simulink model "Final_Project_2"  (R2023b)
settings: Solver=FixedStepAuto  StartTime=0.0  StopTime=inf  FixedStep=0.01  RelTol=1e-3  EnableMultiTasking=on
libraries: arduinolib x8, arduinosensorlib x1
settings Model: ExtModeTrigDuration=2  Creator=FM23  LastModifiedBy=FM23
settings OptimizationCC: EnhancedBackFolding=on  PassReuseOutputArgsAs=Individual arguments  ZeroExternalMemoryAtStartup=off  ZeroInternalMemoryAtStartup=off  MaxStackSize=64  OptimizeBlockOrder=speed  DifferentSizesBufferReuse=on  OptimizationCustomize=off  EfficientTunableParamExpr=on
settings DebuggingCC: ParameterTunabilityLossMsg=error
settings HardwareCC: ProdBitPerInt=16  ProdBitPerPointer=16  ProdBitPerSizeT=16  ProdBitPerPtrDiffT=16  ProdLargestAtomicFloat=None  ProdWordSize=8  ProdHWDeviceType=Atmel->AVR
settings SFSimCC: MATLABDynamicMemAlloc=off
settings RTWCC: Description=Embedded Coder  SystemTargetFile=ert.tlc  HardwareBoard=Arduino Mega 2560  TemplateMakefile=ert_default_tmf  Toolchain=Arduino AVR  BuildConfiguration=Faster Runs
settings CodeAppCC: ForceParamTrailComments=on  IgnoreCustomStorageClasses=off  OperatorAnnotations=on  SimulinkDataObjDesc=on  SFDataObjDesc=on  InsertBlockDesc=on
settings ERTTargetCC: SupportContinuousTime=on  SupportVariableSizeSignals=on  ExtModeTransport=3  ExtModeStaticAlloc=on  ExtModeAutomaticAllocSize=off  ExtModeStaticAllocSize=2048  ExtModeMexFile=ext_xcp  ExtModeIntrfLevel=Level2 - Open

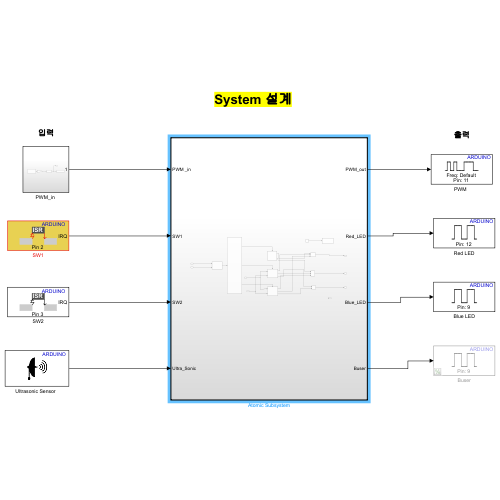
[thumbnail: Simulink's stored preview of the top-level diagram]
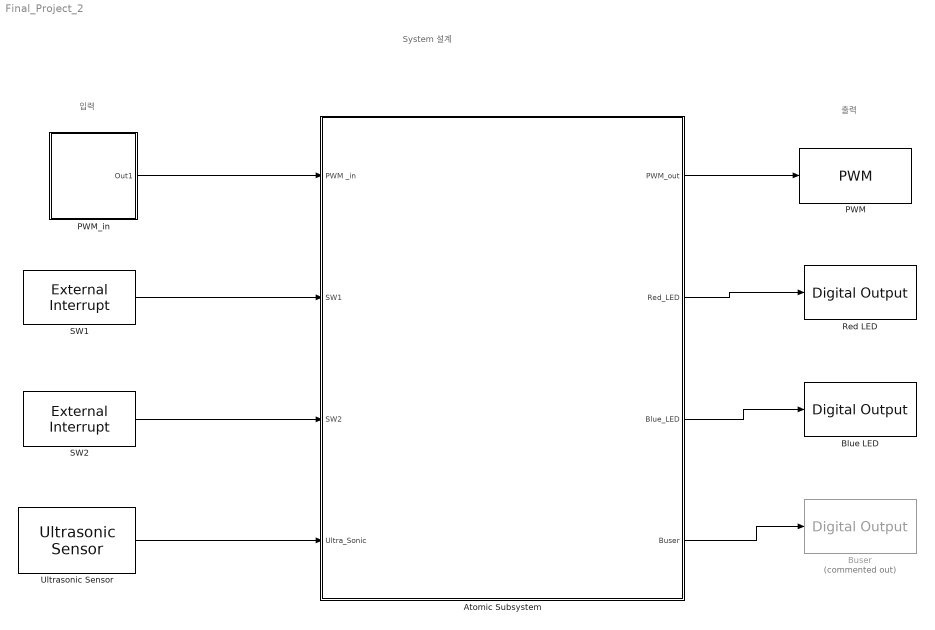
== system Final_Project_2 ==
  note: System 설계
  note: 입력
  note: 출력
  Atomic Subsystem : Subsystem  TreatAsAtomicUnit=on
  Blue LED : arduinolib/Digital Output  pinNumber=9  Direction=output  blockPlatform=arduino
  Buser : arduinolib/Digital Output  Commented=on  pinNumber=9  Direction=output  blockPlatform=arduino
  "PWM  " : arduinolib/PWM  pinNumber=11  frequencyType=Default  desiredFrequency=490.2  achievableFrequency=490.2
  "PWM_in " : Subsystem
  Red LED : arduinolib/Digital Output  pinNumber=12  Direction=output  blockPlatform=arduino
  SW1 : arduinolib/External Interrupt  Pin=2  PullUp=off  Mode=RISING  InterruptSimulationInput=off
  SW2 : arduinolib/External Interrupt  Pin=3  PullUp=off  Mode=RISING  InterruptSimulationInput=off
  "Ultrasonic Sensor  " : arduinosensorlib/Ultrasonic Sensor  NumSignalPins=2  TrigPin=50  EchoPin=51  SignalPin=3  SampleTime_=0.1  blockPlatform=ARDUINO
  wires:
  "Ultrasonic Sensor  "/1 -> Atomic Subsystem/4(Ultra_Sonic)
  "PWM_in "/1(Out1) -> Atomic Subsystem/1(PWM _in)
  Atomic Subsystem/1(" PWM_out") -> "PWM  "/1
  Atomic Subsystem/2(Red_LED) -> Red LED/1
  Atomic Subsystem/3(Blue_LED) -> Blue LED/1
  Atomic Subsystem/4(Buser) -> Buser/1
  SW1/1 -> Atomic Subsystem/2(SW1)
  SW2/1 -> Atomic Subsystem/3(SW2)

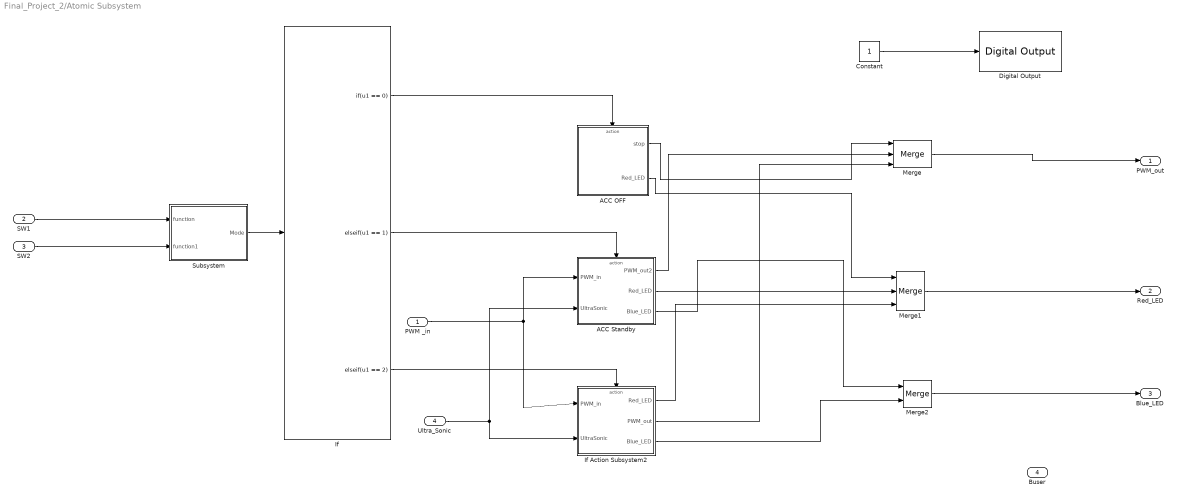
== system Final_Project_2/Atomic Subsystem ==
  PWM _in : Inport
  SW1 : Inport  Port=2
  SW2 : Inport  Port=3
  Ultra_Sonic : Inport  Port=4
  ACC OFF : Subsystem  TreatAsAtomicUnit=on
  "ACC Standby   " : Subsystem  TreatAsAtomicUnit=on
  Constant : Constant
  Digital Output : arduinolib/Digital Output  pinNumber=13  Direction=output  blockPlatform=arduino
  If : If  IfExpression=u1 == 0  ElseIfExpressions=u1 == 1, u1 == 2  ShowElse=off
  If Action Subsystem2 : Subsystem  TreatAsAtomicUnit=on
  Merge : Merge  Inputs=3
  Merge1 : Merge  Inputs=3
  Merge2 : Merge
  Subsystem : Subsystem
  " PWM_out" : Outport
  Red_LED : Outport  Port=2
  Blue_LED : Outport  Port=3
  Buser : Outport  Port=4
  wires:
  Merge1/1 -> Red_LED/1
  Merge2/1 -> Blue_LED/1
  Merge/1 -> " PWM_out"/1
  If/1 -> ACC OFF/Action
  PWM _in/1 -> If Action Subsystem2/1(PWM_in), "ACC Standby   "/1(PWM_in)
  If/2 -> "ACC Standby   "/Action
  ACC OFF/1(stop) -> Merge/1
  If/3 -> If Action Subsystem2/Action
  ACC OFF/2(Red_LED) -> Merge1/1
  "ACC Standby   "/2(Red_LED) -> Merge1/2
  "ACC Standby   "/3(Blue_LED) -> Merge2/1
  "ACC Standby   "/1(PWM_out2) -> Merge/2
  Ultra_Sonic/1 -> If Action Subsystem2/2(UltraSonic), "ACC Standby   "/2(UltraSonic)
  If Action Subsystem2/2(PWM_out) -> Merge/3
  If Action Subsystem2/1(Red_LED) -> Merge1/3
  If Action Subsystem2/3(Blue_LED) -> Merge2/2
  Constant/1 -> Digital Output/1
  Subsystem/1(Mode) -> If/1
  SW1/1 -> Subsystem/1(function)
  SW2/1 -> Subsystem/2(function1)

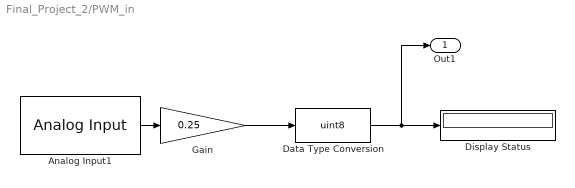
== system Final_Project_2/PWM_in  ==
  Analog Input1 : arduinolib/Analog Input  pinNumber=4  ReadResultsOnly=off  ConversionTriggerSource=Software  ExternalTriggerType=uint32( 0 )  OutputDataType=uint16  EnableConversionCompleteNotify=off  EnableOuputStatus=off  SampleTime=-1  blockPlatform=arduino
  Data Type Conversion : DataTypeConversion  OutDataTypeStr=uint8  SaturateOnIntegerOverflow=off  RndMeth=Floor
  Display Status : Display
  Gain : Gain  Gain=0.25
  Out1 : Outport
  wires:
  Analog Input1/1 -> Gain/1
  Gain/1 -> Data Type Conversion/1
  Data Type Conversion/1 -> Out1/1, Display Status/1

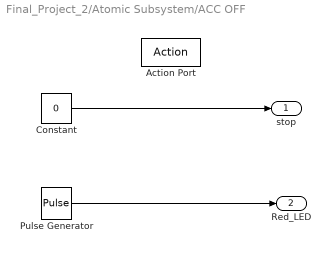
== system Final_Project_2/Atomic Subsystem/ACC OFF ==
  Action Port : ActionPort  ActionPortLabel=if(u1 == 0)
  Constant : Constant  Value=0
  Pulse Generator : DiscretePulseGenerator  PulseType=Time based  Period=10  PulseWidth=5
  stop : Outport
  Red_LED : Outport  Port=2
  wires:
  Constant/1 -> stop/1
  Pulse Generator/1 -> Red_LED/1

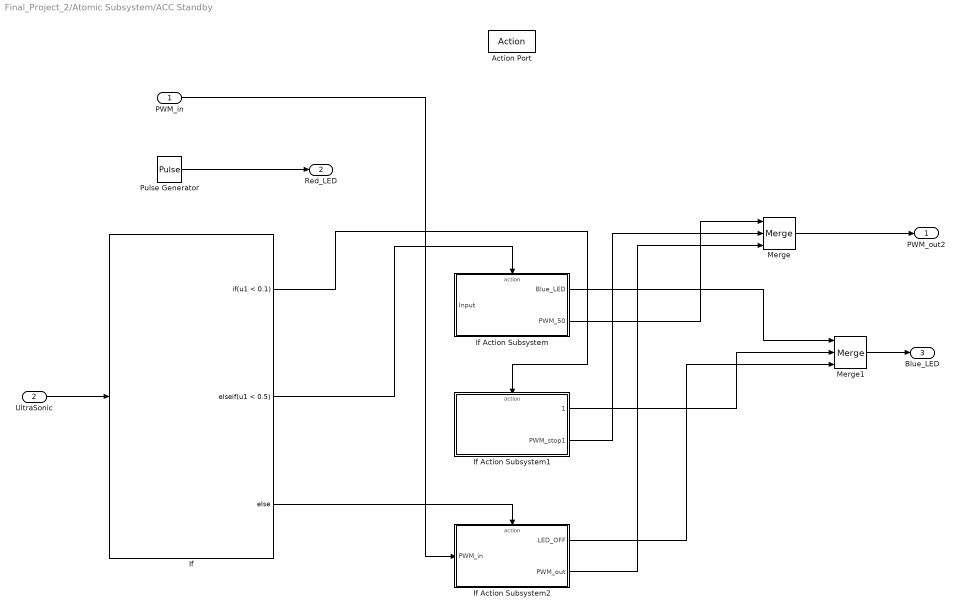
== system Final_Project_2/Atomic Subsystem/ACC Standby    ==
  PWM_in : Inport
  UltraSonic : Inport  Port=2
  Action Port : ActionPort  ActionPortLabel=elseif(u1 == 1)
  If : If  IfExpression=u1 < 0.1  ElseIfExpressions=u1 < 0.5
  If Action Subsystem : Subsystem  TreatAsAtomicUnit=on
  If Action Subsystem1 : Subsystem  TreatAsAtomicUnit=on
  If Action Subsystem2 : Subsystem  TreatAsAtomicUnit=on
  Merge : Merge  Inputs=3
  Merge1 : Merge  Inputs=3
  Pulse Generator : DiscretePulseGenerator  PulseType=Time based  Period=10  PulseWidth=5
  PWM_out2 : Outport
  Red_LED : Outport  Port=2
  Blue_LED : Outport  Port=3
  wires:
  Pulse Generator/1 -> Red_LED/1
  UltraSonic/1 -> If/1
  Merge/1 -> PWM_out2/1
  Merge1/1 -> Blue_LED/1
  If/2 -> If Action Subsystem/Action
  If/1 -> If Action Subsystem1/Action
  If/3 -> If Action Subsystem2/Action
  If Action Subsystem2/2(PWM_out) -> Merge/3
  If Action Subsystem/2(PWM_50) -> Merge/1
  If Action Subsystem/1(Blue_LED) -> Merge1/1
  If Action Subsystem1/1(1) -> Merge1/2
  If Action Subsystem1/2(PWM_stop1) -> Merge/2
  If Action Subsystem2/1(LED_OFF) -> Merge1/3
  PWM_in/1 -> If Action Subsystem2/1(PWM_in)

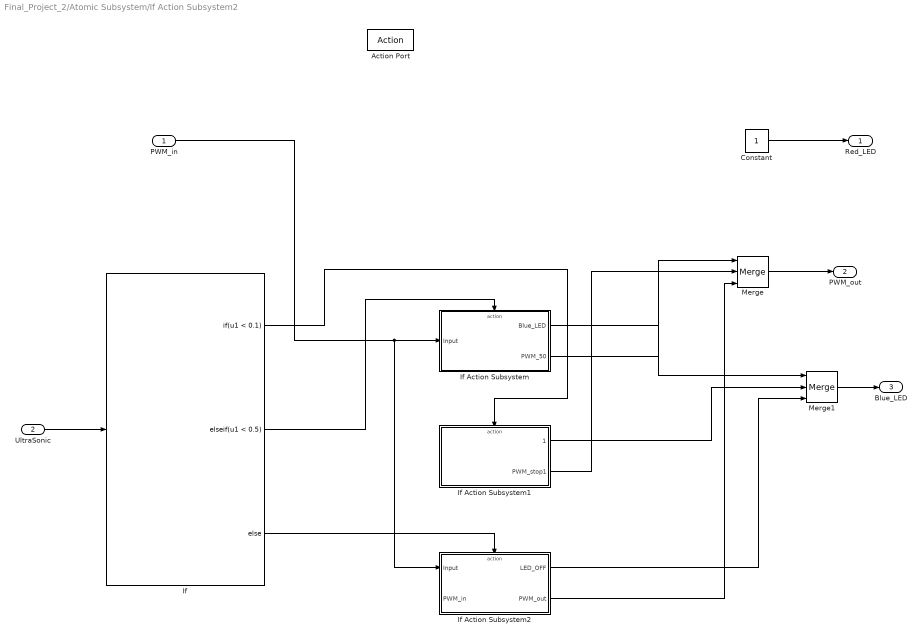
== system Final_Project_2/Atomic Subsystem/If Action Subsystem2 ==
  PWM_in : Inport
  UltraSonic : Inport  Port=2
  Action Port : ActionPort  ActionPortLabel=elseif( u1 == 2)
  Constant : Constant
  If : If  IfExpression=u1 < 0.1  ElseIfExpressions=u1 < 0.5
  If Action Subsystem : Subsystem  TreatAsAtomicUnit=on
  If Action Subsystem1 : Subsystem  TreatAsAtomicUnit=on
  If Action Subsystem2 : Subsystem  TreatAsAtomicUnit=on
  Merge : Merge  Inputs=3
  Merge1 : Merge  Inputs=3
  Red_LED : Outport
  PWM_out : Outport  Port=2
  Blue_LED : Outport  Port=3
  wires:
  If Action Subsystem2/1(LED_OFF) -> Merge1/3
  If Action Subsystem1/2(PWM_stop1) -> Merge/2
  If Action Subsystem2/2(PWM_out) -> Merge/3
  Merge1/1 -> Blue_LED/1
  If Action Subsystem/1(Blue_LED) -> Merge1/1
  If/2 -> If Action Subsystem/Action
  If/3 -> If Action Subsystem2/Action
  If Action Subsystem1/1(1) -> Merge1/2
  If Action Subsystem/2(PWM_50) -> Merge/1
  If/1 -> If Action Subsystem1/Action
  UltraSonic/1 -> If/1
  Merge/1 -> PWM_out/1
  Constant/1 -> Red_LED/1
  PWM_in/1 -> If Action Subsystem2/1(Input), If Action Subsystem/1(Input)

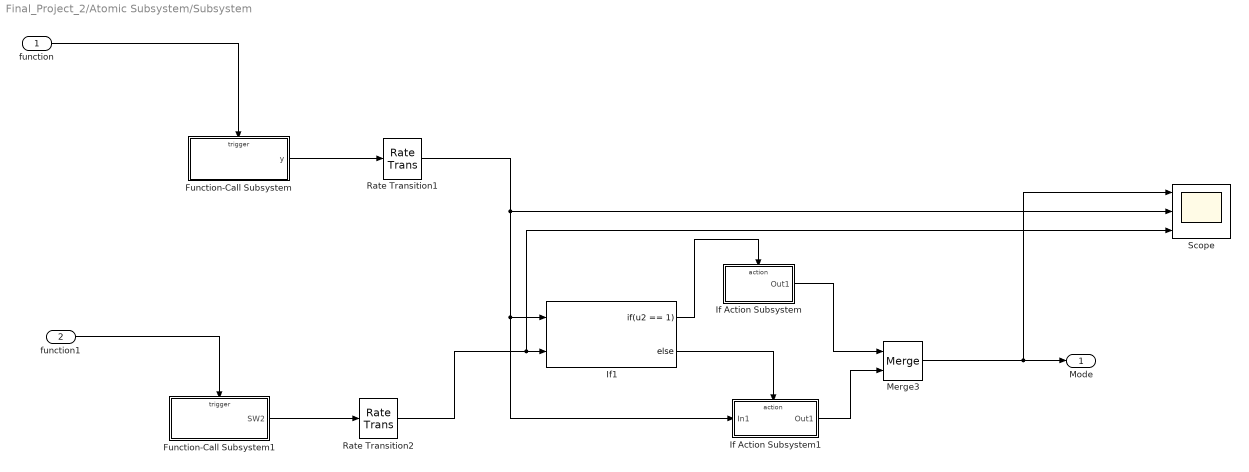
== system Final_Project_2/Atomic Subsystem/Subsystem ==
  function : Inport
  function1 : Inport  Port=2
  Function-Call Subsystem : Subsystem  TreatAsAtomicUnit=on
  Function-Call Subsystem1 : Subsystem  TreatAsAtomicUnit=on
  If Action Subsystem : Subsystem  TreatAsAtomicUnit=on
  If Action Subsystem1 : Subsystem  TreatAsAtomicUnit=on
  If1 : If  NumInputs=2  IfExpression=u2 == 1
  Merge3 : Merge
  Rate Transition1 : RateTransition
  Rate Transition2 : RateTransition
  Scope : Scope  NumInputPorts=3
  Mode : Outport
  wires:
  Merge3/1 -> Mode/1, Scope/1
  If1/1 -> If Action Subsystem/Action
  If Action Subsystem/1(Out1) -> Merge3/1
  function/1 -> Function-Call Subsystem/Trigger
  If1/2 -> If Action Subsystem1/Action
  Function-Call Subsystem1/1(SW2) -> Rate Transition2/1
  If Action Subsystem1/1(Out1) -> Merge3/2
  Rate Transition1/1 -> If Action Subsystem1/1(In1), If1/1, Scope/2
  Rate Transition2/1 -> Scope/3, If1/2
  function1/1 -> Function-Call Subsystem1/Trigger
  Function-Call Subsystem/1(y) -> Rate Transition1/1

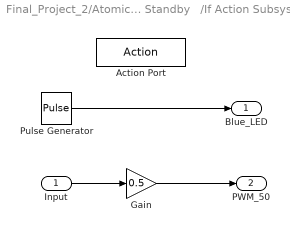
== system Final_Project_2/Atomic Subsystem/ACC Standby   /If Action Subsystem ==
  Input : Inport
  Action Port : ActionPort  ActionPortLabel=elseif(u1 < 0.5)
  Gain : Gain  Gain=0.5
  Pulse Generator : DiscretePulseGenerator  PulseType=Time based  Period=10  PulseWidth=5
  Blue_LED : Outport
  PWM_50 : Outport  Port=2
  wires:
  Pulse Generator/1 -> Blue_LED/1
  Input/1 -> Gain/1
  Gain/1 -> PWM_50/1

== system Final_Project_2/Atomic Subsystem/ACC Standby   /If Action Subsystem1 ==
  Action Port : ActionPort  ActionPortLabel=if(u1 < 0.1)
  Constant : Constant
  Constant1 : Constant  Value=0
  1 : Outport
  PWM_stop1 : Outport  Port=2
  wires:
  Constant/1 -> 1/1
  Constant1/1 -> PWM_stop1/1

== system Final_Project_2/Atomic Subsystem/ACC Standby   /If Action Subsystem2 ==
  PWM_in : Inport
  Action Port : ActionPort  ActionPortLabel=else
  Constant : Constant  Value=0
  LED_OFF : Outport
  PWM_out : Outport  Port=2
  wires:
  Constant/1 -> LED_OFF/1
  PWM_in/1 -> PWM_out/1

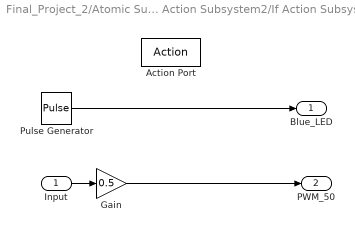
== system Final_Project_2/Atomic Subsystem/If Action Subsystem2/If Action Subsystem ==
  Input : Inport
  Action Port : ActionPort  ActionPortLabel=elseif(u1 < 0.5)
  Gain : Gain  Gain=0.5
  Pulse Generator : DiscretePulseGenerator  PulseType=Time based  Period=10  PulseWidth=5
  Blue_LED : Outport
  PWM_50 : Outport  Port=2
  wires:
  Pulse Generator/1 -> Blue_LED/1
  Input/1 -> Gain/1
  Gain/1 -> PWM_50/1

== system Final_Project_2/Atomic Subsystem/If Action Subsystem2/If Action Subsystem1 ==
  Action Port : ActionPort  ActionPortLabel=if(u1 < 0.1)
  Constant : Constant
  Constant1 : Constant  Value=0
  1 : Outport
  PWM_stop1 : Outport  Port=2
  wires:
  Constant/1 -> PWM_stop1/1
  Constant1/1 -> 1/1

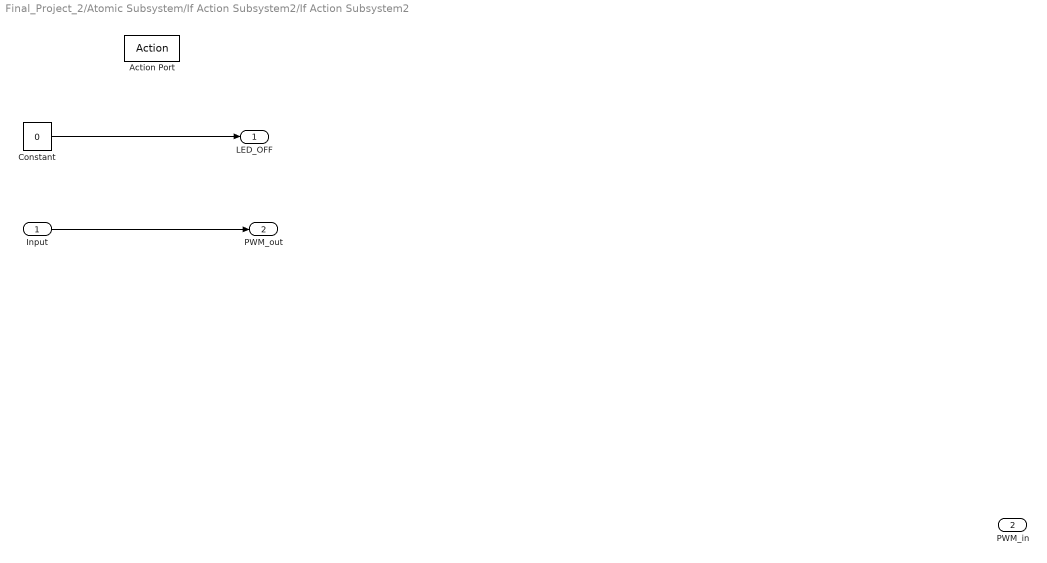
== system Final_Project_2/Atomic Subsystem/If Action Subsystem2/If Action Subsystem2 ==
  Input : Inport
  PWM_in : Inport  Port=2
  Action Port : ActionPort  ActionPortLabel=else
  Constant : Constant  Value=0
  LED_OFF : Outport
  PWM_out : Outport  Port=2
  wires:
  Constant/1 -> LED_OFF/1
  Input/1 -> PWM_out/1

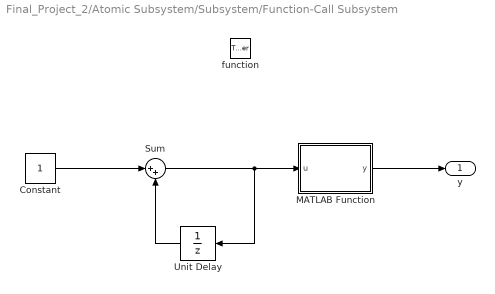
== system Final_Project_2/Atomic Subsystem/Subsystem/Function-Call Subsystem ==
  function : TriggerPort  TriggerType=function-call  VariantControl=(inherit)
  Constant : Constant
  MATLAB Function : MATLAB Function  TreatAsAtomicUnit=on
  Sum : Sum  Inputs=|++
  Unit Delay : UnitDelay  SampleTime=-1  HasFrameUpgradeWarning=on
  y : Outport
  wires:
  Constant/1 -> Sum/1
  Unit Delay/1 -> Sum/2
  Sum/1 -> Unit Delay/1, MATLAB Function/1(u)
  MATLAB Function/1(y) -> y/1

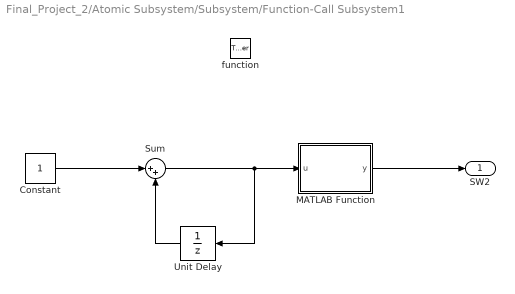
== system Final_Project_2/Atomic Subsystem/Subsystem/Function-Call Subsystem1 ==
  function : TriggerPort  TriggerType=function-call  VariantControl=(inherit)
  Constant : Constant
  MATLAB Function : MATLAB Function  TreatAsAtomicUnit=on
  Sum : Sum  Inputs=|++
  Unit Delay : UnitDelay  SampleTime=-1  HasFrameUpgradeWarning=on
  SW2 : Outport
  wires:
  Constant/1 -> Sum/1
  MATLAB Function/1(y) -> SW2/1
  Unit Delay/1 -> Sum/2
  Sum/1 -> Unit Delay/1, MATLAB Function/1(u)

== system Final_Project_2/Atomic Subsystem/Subsystem/If Action Subsystem ==
  Action Port : ActionPort  ActionPortLabel=if(u2 == 1)
  Constant : Constant  Value=0
  Out1 : Outport
  wires:
  Constant/1 -> Out1/1

== system Final_Project_2/Atomic Subsystem/Subsystem/If Action Subsystem1 ==
  In1 : Inport
  Action Port : ActionPort  ActionPortLabel=else
  Out1 : Outport
  wires:
  In1/1 -> Out1/1

== matlab function Final_Project_2/Atomic Subsystem/Subsystem/Function-Call Subsystem1/MATLAB Function ==
  data: u input; y output
function y = fcn(u)
    % u: 입력 값 (합산기에서 오는 입력)

    % Persistent variable to hold the current state
    persistent state;
   
    % 처음 실행될 때 state를 0으로 초기화
    if isempty(state)
        state = 0;
    end

    % 현재 state 값을 출력
    y = state;
   
    % 다음 state는 0, 1을 순환 (u 값에 관계없이)
    state = mod(state + 1, 2);
end

== matlab function Final_Project_2/Atomic Subsystem/Subsystem/Function-Call Subsystem/MATLAB Function ==
  data: u input; y output
function y = fcn(u)
    % u: 입력 값 (합산기에서 오는 입력)

    % Persistent variable to hold the current state
    persistent state;
   
    % 처음 실행될 때 state를 0으로 초기화
    if isempty(state)
        state = 0;
    end

    % 현재 state 값을 출력
    y = state;
   
    % 다음 state는 0, 1, 2를 순환 (u 값에 관계없이)
    state = mod(state + 1, 3);
end
